simulink model "Microgrid_transition_model_092021"  (R2020a)
settings: Solver=VariableStepAuto  StartTime=0.0  StopTime=10  MaxStep=1e-4  RelTol=1e-3
PreLoadFcn:
  | %run('FC_microgrid_param.m')
  | %load('bat_grid_init.m')
InitFcn:
  | %load myisoModel_init;
  | run('FC_microgrid_param.m')
  | tic
  | run('CARTinitFcn.m')
  | %caseNo = 2;
  | 
  | %if (caseNo == 1)
  | %set_param(['Isolated_grid_paper_model_022521/SignalGen'], 'ActiveScenario', 'PStep222kW');
  | %else
  | %set_param(['Isolated_grid_paper_model_022521/SignalGen'], 'ActiveScenario', 'QStep222kVAr');
  | 
  | %end;
StopFcn:
  | toc
undefined symbols (not defined in the file): breakpoints1, breakpoints2, cp_table_data, ctrl, D1, D11, Delta, DiscIntNeverNeededParam, DT, FC_BESS, find_system, gcbh, libFC_BESS, LowerLimit, magnitude, oversize, pq_ts, sps_rtmsupport, timer, ts, Ts, Ts_APC, Ts_Control, Ts_Power, UpperLimit
libraries: powerlib x128, powerlib_meascontrol x81, simulink x63, powerlib_extras x40, simulink_extras x12, sps_avr x7, pi_ctrl x4, SignalEditorBlockLib x2, libLgBattery x1, libFC_PV x1, eePowerMeasurement x1, spsDieselMotorModel x1
(part 3 of 10)

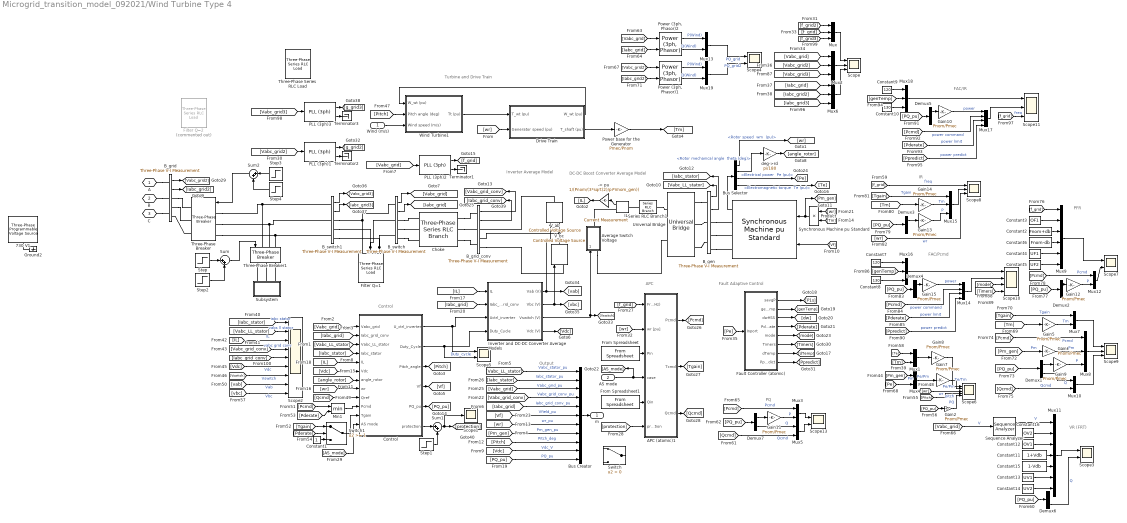
== system Microgrid_transition_model_092021/Wind Turbine Type 4 ==
  note: Control
  note: Turbine and Drive Train
  note: Inverter
      | Average Model
  note: DC-DC Boost Converter
      | Average Model
  note: Fault Adaptive Control
  note: PFR
  note: IR
  note: FAC/Pcmd
  note: PQ
  note: FAC/IR
  note: APC
  note: Output
  note: VR (FRT)
  "Wind (m/s) " : Inport
  AS mode : Inport  Port=2
  -> pu : Gain  Gain=1/(Pnom/(3*sqrt(2)/pi*Vnom_gen))  SaturateOnIntegerOverflow=on  OutDataTypeStr=Inherit: Same as input  ParamDataTypeStr=Inherit: Same as input
  730 V1 : powerlib/Electrical Sources/Three-Phase Programmable Voltage Source  PositiveSequence=[730 0 60]  VariationEntity=None  VariationType=Table of time-amplitude pairs  VariationTypeAlt=Step  VariationStep=-0.2  VariationRate=10  VariationMagnitude=0.3  VariationFrequency=2  VariationTiming=[0.05 0.05+5/60]  VariationPhaseA=off  Amplitudes=[1 1 1.0]  TimeValues=[0 0.03 0.13]  HarmonicGeneration=off  HarmonicA=[1 -0.1 0 2]  HarmonicB=[2 0.15 35 2]*0  Timing="[0.1  2]"  BusType=swing  Pref=0  Qref=0  Qmin=-inf  Qmax=inf
  APC (atomic)1 : Subsystem  TreatAsAtomicUnit=on  SystemSampleTime=0.01
  Average Switch Voltage : Subsystem
  B_gen : powerlib/Measurements/Three-Phase V-I Measurement  VoltageMeasurement=phase-to-phase  SetLabelV=off  LabelV=Vabc  Vpu=on  VpuLL=off  CurrentMeasurement=yes  SetLabelI=off  LabelI=Iabc  Ipu=on  Pbase=Pnom  Vbase=Vnom_gen  OutputType=Complex  PhasorSimulation=off  PSBequivalent=0
      settings: SourceProductBaseCode=MT,PS
  B_grid : powerlib/Measurements/Three-Phase V-I Measurement  VoltageMeasurement=phase-to-ground  SetLabelV=off  LabelV=Vabc  Vpu=on  VpuLL=off  CurrentMeasurement=yes  SetLabelI=off  LabelI=Iabc  Ipu=on  Pbase=Pnom  Vbase=Vnom  OutputType=Complex  PhasorSimulation=off  PSBequivalent=0
      settings: SourceProductBaseCode=MT,PS
  B_grid_conv : powerlib/Measurements/Three-Phase V-I Measurement  VoltageMeasurement=phase-to-ground  SetLabelV=off  LabelV=Vabc  Vpu=on  VpuLL=off  CurrentMeasurement=yes  SetLabelI=off  LabelI=Iabc  Ipu=on  Pbase=Pnom  Vbase=Vnom  OutputType=Complex  PhasorSimulation=off  PSBequivalent=0
      settings: SourceProductBaseCode=MT,PS
  B_switch : powerlib/Measurements/Three-Phase V-I Measurement  VoltageMeasurement=phase-to-ground  SetLabelV=off  LabelV=Vabc  Vpu=on  VpuLL=off  CurrentMeasurement=yes  SetLabelI=off  LabelI=Iabc  Ipu=on  Pbase=Pnom  Vbase=Vnom  OutputType=Complex  PhasorSimulation=off  PSBequivalent=0
      settings: SourceProductBaseCode=MT,PS
  B_switch1 : powerlib/Measurements/Three-Phase V-I Measurement  VoltageMeasurement=phase-to-ground  SetLabelV=off  LabelV=Vabc  Vpu=on  VpuLL=off  CurrentMeasurement=yes  SetLabelI=off  LabelI=Iabc  Ipu=on  Pbase=Pnom  Vbase=Vnom  OutputType=Complex  PhasorSimulation=off  PSBequivalent=0
      settings: SourceProductBaseCode=MT,PS
  Bus Creator : BusCreator  Inputs=11
  Bus Selector : BusSelector  OutputSignals="Mechanical.Rotor speed  wm  (pu),Mechanical.Rotor mechanical angle  theta (deg),Mechanical.Electrical power  Pe (pu),Mechanical.Electromagnetic torque  Te (pu)"
  "Choke " : powerlib/Elements/Three-Phase Series RLC Branch  LConnTagsString=A|B|C  RConnTagsString=A|B|C  BranchType=RL  Resistance=R_RL*Vnom^2/Pnom  Inductance=L_RL*Vnom^2/Pnom/(2*pi*Fnom)  Capacitance=[]  Measurements=None
      settings: SourceProductBaseCode=MT,PS
  Constant1 : Constant
  Constant10 : Constant  Value=130
  Constant11 : Constant  Value=1+Vdb
  Constant12 : Constant  Value=OV1
  Constant13 : Constant  Value=UV1
  Constant14 : Constant  Value=UV2
  Constant15 : Constant  Value=1-Vdb
  Constant16 : Constant  Value=OV2
  Constant2 : Constant  Value=Fnom+db
  Constant3 : Constant  Value=OF1
  Constant4 : Constant  Value=UF1
  Constant5 : Constant  Value=UF2
  Constant6 : Constant  Value=Fnom-db
  Constant7 : Constant  Value=120
  Constant8 : Constant  Value=130
  Constant9 : Constant  Value=120
  Control : Subsystem
  Demux{1..7} (7 alike) : Demux  Outputs=2
  Drive Train : Subsystem  mask(Wind Turbine shaft){H_WT=H_WT/10, Ksh=Ksh, D_mutual=D_mutual, wbase=2*pi*Fnom/p, w_wt0=w_wt0, torque0=torque0, Ts=Ts}
      mask prompts: H_WT "Wind turbine inertia constant H (s):"; Ksh "Shaft spring constant (pu of nominal mechanical torque/rad):"; D_mutual "Shaft mutual damping (pu of nominal mechanical torque/pu dw):"; wbase "Shaft base speed (rad/s):"; w_wt0 "Turbine initial speed (pu of base speed):"; torque0 "Initial output torque (pu of nominal mechanical torque):"; Ts "Sample time (s):"
      mask help:
      | This block implements a wind turbine drive train model. All shaft parameters are referred to high-speed shaft (generator shaft).
      |
      | The first input is the wind turbine torque in per unit (pu) based on the nominal power of the turbine and the base speed of the generator. The second input is the generator speed in pu based on the base speed of the generator.
      |
      | The outputs are:
      | 1- the transmitted torque of the shaft in pu based on the nominal power of the turbine and the base speed of the generator.
      | 2- the wind turbine speed in pu of the base speed of the generator.
  "Fault Controller (atomic) " : Subsystem  TreatAsAtomicUnit=on  SystemSampleTime=Ts_APC
  Filter Q=1 : powerlib/Elements/Three-Phase Series RLC Load  LConnTagsString=A|B|C  Configuration=Y (grounded)  NominalVoltage=Vnom  Vabc=[1e3 1e3 1e3]  Vabcp=[1e3 1e3 1e3]  NominalFrequency=Fnom  UnbalancedPower=off  ActivePower=100  InductivePower=100  CapacitivePower=100  Pabc=[10e3 9e3 11e3]  QLabc=[100 90 110]  QCabc=[100 90 110]  Pabcp=[10e3 9e3 11e3]  QLabcp=[100 90 110]  QCabcp=[100 90 110]  Measurements=None  LoadType=constant Z
      settings: SourceProductBaseCode=MT,PS
  Filter Q=2 : powerlib/Elements/Three-Phase Series RLC Load  Commented=on  LConnTagsString=A|B|C  Configuration=Y (grounded)  NominalVoltage=Vnom  Vabc=[1e3 1e3 1e3]  Vabcp=[1e3 1e3 1e3]  NominalFrequency=Fnom  UnbalancedPower=off  ActivePower=C_var_filter/Q_filter  InductivePower=0  CapacitivePower=C_var_filter  Pabc=[10e3 9e3 11e3]  QLabc=[100 90 110]  QCabc=[100 90 110]  Pabcp=[10e3 9e3 11e3]  QLabcp=[100 90 110]  QCabcp=[100 90 110]  Measurements=None  LoadType=constant Z
      settings: SourceProductBaseCode=MT,PS
  From Spreadsheet : FromSpreadsheet  FileName=Microgrid_cmd.xlsx  SheetName=P  SampleTime=Ts_APC
  From Spreadsheet1 : FromSpreadsheet  FileName=Microgrid_cmd.xlsx  SheetName=Q  SampleTime=Ts_APC
  Gain{2,5..15} (12 alike) : Gain  Gain=Pnom/Pmec
  Ground2 : powerlib/Elements/Ground  LConnTagsString=a
  IL : powerlib/Measurements/Current Measurement  PhasorSimulation=off  OutputType=Complex  PSBequivalent=0
      settings: SourceProductBaseCode=MT,PS
  Inverter and DC-DC Converter Average Models : Subsystem
  Min1 : MinMax  Inputs=2
  Mux{,2,6,8,15..16,18} (7 alike) : Mux  Inputs=3
  Mux{1,3..5,7,10,12..13,19} (9 alike) : Mux  Inputs=2
  Mux11 : Mux  Inputs=7
  Mux14 : Mux
  Mux17 : Mux
  Mux9 : Mux  Inputs=6
  PLL (3ph)1 : powerlib_meascontrol/PLL/PLL (3ph)  Fmin=45  Par_Init=[0, 60]  ParK=[180, 3200, 1]  TcD=1e-4  MaxRateChangeFreq=12  FilterCutOffFreq=25  Ts=Ts  AGC=on
  PLL (3ph)2 : powerlib_meascontrol/PLL/PLL (3ph)  Fmin=45  Par_Init=[0, 60]  ParK=[180, 3200, 1]  TcD=1e-4  MaxRateChangeFreq=12  FilterCutOffFreq=25  Ts=Ts  AGC=on
  PLL (3ph)3 : powerlib_meascontrol/PLL/PLL (3ph)  Fmin=45  Par_Init=[0, 60]  ParK=[180, 3200, 1]  TcD=1e-4  MaxRateChangeFreq=12  FilterCutOffFreq=25  Ts=Ts  AGC=on
  "Power (3ph, Phasor)1" : powerlib_meascontrol/Measurements/Power (3ph, Phasor)
      settings: SourceProductBaseCode=PS
  "Power (3ph, Phasor)2" : powerlib_meascontrol/Measurements/Power (3ph, Phasor)
      settings: SourceProductBaseCode=PS
  Power base for the Generator : Gain  Gain=Pmec/Pnom  SaturateOnIntegerOverflow=on  OutDataTypeStr=Inherit: Same as input  ParamDataTypeStr=Inherit: Same as input
  Product : Product  RndMeth=Zero
  Scope{,8..9,11} (4 alike) : Scope  NumInputPorts=3
  Scope1 : Scope
  Scope10 : Scope  NumInputPorts=4
  Scope{3..5,7,13} (5 alike) : Scope  NumInputPorts=2
  Scope2 : Scope  NumInputPorts=9
  Scope6 : Scope  NumInputPorts=5
  Sequence Analyzer : powerlib_meascontrol/Measurements/Sequence Analyzer  Freq=60  n=1  seq=Positive  InInit=[1, 0]  Ts=Ts
      settings: SourceProductBaseCode=PS
  Series RLC Branch1 : powerlib/Elements/Series RLC Branch  LConnTagsString=__new0  RConnTagsString=__new0  BranchType=RL  Resistance=R_Boost  Inductance=L_Boost  SetiL0=off  InitialCurrent=0  Capacitance=1.0  Setx0=off  InitialVoltage=0  Measurements=Branch current
      settings: SourceProductBaseCode=MT,PS
  Step : Step  Time=4  Before=1  After=0  SampleTime=Ts
  Step1 : Step  Time=99  After=0  SampleTime=Ts
  Step2 : Step  Time=3  SampleTime=Ts
  Step3 : Step  Time=3  Before=1  After=0  SampleTime=Ts
  Step4 : Step  Time=4  SampleTime=Ts
  Subsystem : Subsystem
  Sum : Sum  Inputs=|++
  Sum1 : Sum  Inputs=|++
  Sum2 : Sum  Inputs=|++
  Switch : Switch  Criteria=u2 > Threshold
  Switch1 : Switch  Threshold=1
  Synchronous Machine pu Standard : powerlib/Machines/Synchronous Machine pu Standard  PresetModel=No  MechanicalLoad=Mechanical power Pm  ShowDetailedParameters=on  RotorType=Salient-pole  Units=per unit standard parameters  MeasurementBus=off  NominalParameters="[ Pnom  Vnom_gen Fnom ]"  Reactances1=[ 1.81, 0.3, 0.23, 1.76, 0.65, 0.25, 0.15 ]  Reactances2="[ Xd, Xd1, Xd2, Xq,  Xq2,  Xl ]"  dAxisTimeConstants=Open-circuit  qAxisTimeConstants=Short-circuit  TimeConstants1="[ 4.4849  0.0681  0.1  ]"  TimeConstants2=[ 8.0, 0.03, 1.0, 0.07 ]  TimeConstants3="[  Tdo1  Tdo2  Tq2  ]"  TimeConstants4=[ 8.0, 0.03, 0.3371, 0.0295 ]  TimeConstants5=[ 1.01, 0.053, 0.1 ]  TimeConstants6=[ 1.3201, 0.023, 1.0, 0.07 ]  TimeConstants7="[  1.01  0.053  0.051266  ]"  TimeConstants8=[ 1.3201, 0.0231, 0.3371, 0.0295 ]  StatorResistance=Resistance  Mechanical=[ H F p]  PolePairs=1  InitialConditions=init  SetSaturation=off  Saturation=[0.6404,0.7127,0.8441,0.9214,0.9956,1.082,1.19,1.316,1.457;0.7,0.7698,0.8872,0.9466,0.9969,1.046,1.1,1.151,1.201]  LoadFlowParameters=[1,0,0,0,0]  TsPowergui=0  TsBlock=-1  IterativeModel=Trapezoidal non iterative  IterativeDiscreteModel=Trapezoidal non iterative  BusType=PV  Pref=0  Qref=0  Qmin=-inf  Qmax=inf  PLF=0  QLF=0
      settings: SourceProductBaseCode=MT,PS
  Terminator1 : Terminator
  Terminator2 : Terminator
  Terminator3 : Terminator
  Three-Phase Series RLC Load : powerlib/Elements/Three-Phase Series RLC Load  LConnTagsString=A|B|C  Configuration=Y (grounded)  NominalVoltage=1000  Vabc=[1e3 1e3 1e3]  Vabcp=[1e3 1e3 1e3]  NominalFrequency=60  UnbalancedPower=off  ActivePower=10e3  InductivePower=100  CapacitivePower=100  Pabc=[10e3 9e3 11e3]  QLabc=[100 90 110]  QCabc=[100 90 110]  Pabcp=[10e3 9e3 11e3]  QLabcp=[100 90 110]  QCabcp=[100 90 110]  Measurements=None  LoadType=constant Z
  Three-Phase Breaker : powerlib/Elements/Three-Phase Breaker  InitialState=closed  SwitchA=on  SwitchB=on  SwitchC=on  SwitchTimes=[1000]  External=on  BreakerResistance=Ron_breaker/Nb_WT  SnubberResistance=Rs_breaker/Nb_WT  SnubberCapacitance=Cs_breaker*Nb_WT  Measurements=None
  Three-Phase Breaker1 : powerlib/Elements/Three-Phase Breaker  InitialState=closed  SwitchA=on  SwitchB=on  SwitchC=on  SwitchTimes=[1000]  External=on  BreakerResistance=Ron_breaker/Nb_WT  SnubberResistance=Rs_breaker/Nb_WT  SnubberCapacitance=Cs_breaker*Nb_WT  Measurements=None
  Universal Bridge : powerlib/Power Electronics/Universal Bridge  Arms=3  SnubberResistance=2*Ts_snub/(Pnom/(1000*2*pi*Fnom*Vnom_gen^2))  SnubberCapacitance=Pnom/(1000*2*pi*Fnom*Vnom_gen^2)  Device=Diodes  Ron=1e-6/Nb_wt  Lon=0  ForwardVoltages="[  0  0  ]"  ForwardVoltage=0  GTOparameters=[ 10e-6 , 20e-6 ]  IGBTparameters=[ 1e-6 , 2e-6 ]  Measurements=None  Measurements_2=None  converterType=Rectifier
      settings: SourceProductBaseCode=MT,PS
  V_ab : powerlib/Electrical Sources/Controlled Voltage Source  Initialize=on  Source_Type=AC  Amplitude=0  Phase=0  Frequency=0  Measurements=None
      settings: SourceProductBaseCode=MT,PS
  V_bc : powerlib/Electrical Sources/Controlled Voltage Source  Initialize=on  Source_Type=AC  Amplitude=0  Phase=0  Frequency=0  Measurements=None
      settings: SourceProductBaseCode=MT,PS
  Wind Turbine1 : Subsystem  mask(Wind Turbine){Prated=Pmec, c1_c8=c1_c8, K1_K2=K1_K2, wind0=wind0, Ts=Ts}
      mask prompts: Prated "Nominal mechanical output power (W):"; c1_c8 "Coefficients [c1 ... c8]"; K1_K2 "Parameters [K1 K2]"; wind0 "Initial wind speed (m/s):"; Ts "Sample time (s):"
      mask help:
      | This block implements a generic wind turbine models.
      |
      | The first input is the turbine speed in per unit of the generator base speed. For a synchronous or asynchronous generator, the base speed is the synchronous speed. For a permanent-magnet generator, the base speed is defined as the speed producing nominal voltage at  no load. The second input is the blade pitch angle in degrees. The third input is the wind speed in m/s.
      |
      | The output is the torque applied to the drive train in per unit based on the nominal power of the turbine and the base speed of the generator.
      mask init:
      | c1 = c1_c8(1);
      | c2 = c1_c8(2);
      | c3 = c1_c8(3);
      | c4 = c1_c8(4);
      | c5 = c1_c8(5);
      | c6 = c1_c8(6);
      | c7 = c1_c8(7);;
      | c8 = c1_c8(8);
      | 
      | K1=K1_K2(1);
      | K2=K1_K2(2);
      settings: OpenFcn=power_openblockproxy();
      mask Display: disp('');
  deg->rd : Gain  Gain=pi/180  SaturateOnIntegerOverflow=on  OutDataTypeStr=Inherit: Same as input  ParamDataTypeStr=Inherit: Same as input
  A : PMIOPort  Tag=PMCPort  Side=Left
  B : PMIOPort  Tag=PMCPort  Port=2  Side=Left
  C : PMIOPort  Tag=PMCPort  Port=3  Side=Left
  m : Outport  VectorParamsAs1DForOutWhenUnconnected=off
  wires:
  Bus Selector/2 -> deg->rd/1  "<Rotor mechanical angle  theta (deg)>"
  deg->rd/1 -> [angle_rotor]
  Bus Selector/1 -> [wr]  "<Rotor speed  wm  (pu)>"
  [Iabc_grid] -> Inverter and DC-DC Converter Average Models/2(Iabc_grid_conv)
  [IL] -> Inverter and DC-DC Converter Average Models/1(IL)
  [Vabc_grid] -> Control/1(Vabc_grid)
  [Iabc_grid] -> Control/2(Iabc_grid_conv)
  [Vabc_LL_stator] -> Control/3(Vabc_LL_stator)
  [Iabc_stator] -> Control/4(Iabc_stator)
  [Vdc] -> Control/6(Vdc)
  [angle_rotor] -> Control/7(angle_rotor)
  [wr] -> Control/8(wr)
  Control/2(Duty_Cycle) -> Scope5/2, Inverter and DC-DC Converter Average Models/4(Duty_Cycle)  "Duty_cycle"
  Control/3(Pitch_angle) -> [Pitch]
  Control/4(Vf) -> [Vf]
  Control/5(PQ_pu) -> [PQ_pu]
  [IL] -> Control/5(IL)
  Control/1(U_ctrl_inverter) -> Scope5/1, Inverter and DC-DC Converter Average Models/3(Uctrl_inverter)
  Inverter and DC-DC Converter Average Models/4(Vdc (V)) -> [Vdc]
  [Qcmd] -> Control/9(Qref)
  [Pitch] -> Wind Turbine1/2(Pitch angle (deg))
  Drive Train/2(T_shaft (pu)) -> Power base for the Generator/1
  Drive Train/1(W_wt (pu)) -> Wind Turbine1/1(W_wt (pu))
  "Wind (m/s) "/1 -> Wind Turbine1/3(Wind speed (m/s))
  Power base for the Generator/1 -> [Tm]
  [wr] -> Drive Train/2(Generator speed (pu))
  Wind Turbine1/1(Tt (pu)) -> Drive Train/1(T_wt (pu))
  Bus Selector/4 -> [Te]  "<Electromagnetic torque  Te (pu)>"
  Bus Selector/3 -> [Pe]  "<Electrical power  Pe (pu)>"
  Inverter and DC-DC Converter Average Models/1(Vab (V)) -> V_ab/1, [vab]
  [wr] -> Product/1
  B_gen/2 -> [Iabc_stator]
  Inverter and DC-DC Converter Average Models/2(Vbc (V)) -> V_bc/1, [vbc]
  B_switch/2 -> [Iabc_grid]
  Synchronous Machine pu Standard/1 -> Bus Selector/1
  B_switch/1 -> [Vabc_grid]
  [Tm] -> Product/2
  IL/1 -> -> pu/1
  B_gen/1 -> [Vabc_LL_stator]
  [Vf] -> Synchronous Machine pu Standard/2
  Inverter and DC-DC Converter Average Models/3(Vswitch (V)) -> Average Switch Voltage/1(Vswitch), [Vswitch]
  B_grid_conv/1 -> [Vabc_grid_conv]
  Product/1 -> Synchronous Machine pu Standard/1, [Pm_gen]
  -> pu/1 -> [IL]
  Control/6(protection) -> Sum1/1
  "Fault Controller (atomic) "/1(savgP) -> [P1s]
  [Pe] -> "Fault Controller (atomic) "/1(Inport)
  "Fault Controller (atomic) "/8(Ppredict) -> [Ppredict]
  "Fault Controller (atomic) "/2(genTemp) -> [genTemp]
  "Fault Controller (atomic) "/7(dTemp) -> [dTemp]
  "Fault Controller (atomic) "/6(Timers) -> [Timers]
  "Fault Controller (atomic) "/4(Pderate) -> [Pderate]
  "Fault Controller (atomic) "/3(dwHSS) -> [dw]
  "Fault Controller (atomic) "/5(mode) -> [mode]
  Gain8/1 -> Scope6/1  "Te/Tm"
  [Tm] -> Gain14/1
  [PQ_pu] -> Demux2/1
  [Tm] -> Mux1/2
  Constant10/1 -> Mux18/3
  [Qcmd] -> Mux10/2  "Qcmd"
  Mux12/1 -> Scope7/2
  [Pcmd] -> Mux8/1  "Pcmd"
  [Te] -> Mux1/1
  Mux9/1 -> Scope7/1
  [PQ_pu] -> Demux4/1
  Gain13/1 -> Mux15/3  "P"
  Gain14/1 -> Mux15/2  "Tm"
  Gain12/1 -> Mux12/2  "P"
  [Tgain] -> Mux7/1  "Tgain"
  Demux5/1 -> Gain10/1
  Gain9/1 -> Mux8/3  "P"
  [Pderate] -> Mux14/3  "power limit"
  [Pe] -> Mux4/2
  [wr] -> Scope8/3  "wr"
  Mux17/1 -> Scope11/2
  Demux1/1 -> Gain9/1
  [Timers] -> Scope10/4
  Mux5/1 -> Scope13/2
  Mux4/1 -> Gain7/1  "Pe/Pm"
  [f_grid] -> Scope8/1  "freq"
  [Ppredict] -> Mux14/4  "power predict"
  Mux10/1 -> Scope9/3
  Demux1/2 -> Mux10/1  "Q"
  [Pm_gen] -> Mux4/1  "Pm"
  [genTemp] -> Mux18/2
  [Pitch] -> Scope6/4  "pitch"
  Mux14/1 -> Scope10/2
  [PQ_pu] -> Gain2/1
  Constant9/1 -> Mux18/1
  Constant8/1 -> Mux16/3
  [PQ_pu] -> Demux1/1
  [Pderate] -> Mux17/3  "power limit"
  [Pcmd] -> Mux17/2  "power command"
  Mux1/1 -> Gain8/1
  Mux8/1 -> Scope9/2
  Gain15/1 -> Mux14/1  "power"
  Constant2/1 -> Mux9/3
  Mux16/1 -> Scope10/1
  [Pcmd] -> Mux14/2  "power command"
  [Pcmd] -> Mux12/1  "Pcmd"
  Constant7/1 -> Mux16/1
  Mux15/1 -> Scope8/2
  [PQ_pu] -> Demux5/1
  Gain11/1 -> Mux3/2  "P"
  Gain5/1 -> Mux7/2  "Tm"
  [Pm_gen] -> Gain6/1  "Pm"
  [PQ_pu] -> Demux7/1
  [f_grid] -> Scope11/3  "freq"
  Gain10/1 -> Mux17/1  "power"
  [Tgain] -> Mux15/1  "Tgain"
  Gain6/1 -> Mux8/2  "Pm"
  [Qcmd] -> Mux5/2  "Qcmd"
  [Tm] -> Gain5/1
  [wr] -> Scope6/3  "wr"
  Mux3/1 -> Scope13/1
  Demux2/1 -> Gain12/1
  Demux4/1 -> Gain15/1
  Constant3/1 -> Mux9/2
  Constant5/1 -> Mux9/6
  Demux7/2 -> Mux5/1  "Q"
  [PQ_pu] -> Demux3/1
  [Pcmd] -> Mux3/1  "Pcmd"
  [Ppredict] -> Mux17/4  "power predict"
  Constant6/1 -> Mux9/4
  Demux3/1 -> Gain13/1
  Constant4/1 -> Mux9/5
  Gain2/1 -> Scope6/5  "PQ"
  Demux7/1 -> Gain11/1
  Mux18/1 -> Scope11/1
  Mux7/1 -> Scope9/1
  [f_grid] -> Mux9/1
  Gain7/1 -> Scope6/2  "Pe/Pm"
  [mode] -> Scope10/3
  [genTemp] -> Mux16/2
  [Pderate] -> Min1/2
  [Pcmd] -> Min1/1
  Min1/1 -> Control/10(Pcmd)
  [Pderate] -> Switch1/2
  Switch1/1 -> Control/11(Tgain)
  Constant1/1 -> Switch1/3
  [Tgain] -> Switch1/1
  PLL (3ph)2/2 -> Terminator1/1
  [Vabc_grid] -> PLL (3ph)2/1
  PLL (3ph)2/1 -> [f_grid]
  From Spreadsheet1/1 -> APC (atomic)1/5(Qin)
  [f_grid] -> APC (atomic)1/1(Freq (Hz))
  APC (atomic)1/3(Qcmd) -> [Qcmd]
  APC (atomic)1/2(Tcmd) -> [Tgain]
  [protection] -> APC (atomic)1/6(protection)
  [wr] -> APC (atomic)1/2(wr [pu])
  AS mode/1 -> APC (atomic)1/4(case), [AS_mode]
  APC (atomic)1/1(Pcmd) -> [Pcmd]
  From Spreadsheet/1 -> APC (atomic)1/3(Pin)
  [AS_mode] -> Control/12(AS mode)
  [Pm_gen] -> Bus Creator/8  "Pm_gen_pu"
  Bus Creator/1 -> m/1
  [Iabc_grid] -> Bus Creator/5  "Iabc_grid_conv_pu"
  [Pitch] -> Bus Creator/9  "Pitch_deg"
  [PQ_pu] -> Bus Creator/11  "PQ_pu"
  [Vf] -> Bus Creator/6  "Vfield_pu"
  [Vdc] -> Bus Creator/10  "Vdc_V"
  [Vabc_LL_stator] -> Bus Creator/1  "Vabc_stator_pu"
  [Vabc_grid] -> Bus Creator/3  "Vabc_grid_pu"
  [Iabc_stator] -> Bus Creator/2  "Iabc_stator_pu"
  [wr] -> Bus Creator/7  "wr_pu"
  [Vabc_grid_conv] -> Bus Creator/4  "Vabc_grid_conv_pu"
  B_grid/2 -> [Iabc_grid2]
  B_grid/1 -> [Vabc_grid2]
  PLL (3ph)1/1 -> [g_grid2]
  PLL (3ph)1/2 -> Terminator2/1
  [Vabc_grid2] -> PLL (3ph)1/1
  [f_grid2] -> Mux/1
  [f_grid] -> Mux/2
  [Vabc_grid] -> Mux2/1
  [Vabc_grid2] -> Mux2/2
  Mux2/1 -> Scope/2
  Mux/1 -> Scope/1
  Sum2/1 -> Three-Phase Breaker/1
  Step1/1 -> Sum1/2
  Sum1/1 -> [protection], Scope1/1
  [Iabc_stator] -> Scope2/1  "iabc stator"
  [Vabc_LL_stator] -> Scope2/2  "vabs ll stator"
  [IL] -> Scope2/3  "IL"
  [Vabc_grid_conv] -> Scope2/4  "vabc grid conv"
  [Vdc] -> Scope2/6  "Vdc"
  [Vswitch] -> Scope2/7  "Vswitch"
  [vab] -> Scope2/8  "Vab"
  [vbc] -> Scope2/9  "Vbc"
  Sequence Analyzer/1 -> Mux11/1  "V"
  Constant13/1 -> Mux11/6
  Constant15/1 -> Mux11/5
  Constant14/1 -> Mux11/7
  Constant12/1 -> Mux11/3
  Constant11/1 -> Mux11/4
  Mux11/1 -> Scope3/1
  [Vabc_grid] -> Sequence Analyzer/1  "V"
  Constant16/1 -> Mux11/2
  Demux6/2 -> Scope3/2  "Q"
  [PQ_pu] -> Demux6/1
  "Power (3ph, Phasor)2"/2 -> Mux13/2  "Q(Wind)"
  [Vabc_grid] -> "Power (3ph, Phasor)2"/1
  "Power (3ph, Phasor)2"/1 -> Mux13/1  "P(Wind)"
  [Iabc_grid] -> "Power (3ph, Phasor)2"/2
  Mux13/1 -> Scope4/1  "PQ_grid"
  Mux19/1 -> Scope4/2  "PQ_grid2"
  [Iabc_grid2] -> "Power (3ph, Phasor)1"/2
  [Vabc_grid2] -> "Power (3ph, Phasor)1"/1
  "Power (3ph, Phasor)1"/1 -> Mux19/1  "P(Wind)"
  "Power (3ph, Phasor)1"/2 -> Mux19/2  "Q(Wind)"
  B_switch1/1 -> [Vabc_grid3]
  B_switch1/2 -> [Iabc_grid3]
  PLL (3ph)3/1 -> [g_grid3]
  PLL (3ph)3/2 -> Terminator3/1
  [Vabc_grid3] -> PLL (3ph)3/1
  [f_grid3] -> Mux/3
  [Vabc_grid3] -> Mux2/3
  [Iabc_grid] -> Mux6/1
  [Iabc_grid2] -> Mux6/2
  [Iabc_grid3] -> Mux6/3
  Mux6/1 -> Scope/3
  B_grid_conv/2 -> [Iabc_grid_conv]
  [Iabc_grid_conv] -> Scope2/5
  Step2/1 -> Sum/2
  Step/1 -> Sum/1
  Sum/1 -> Three-Phase Breaker1/1
  Step4/1 -> Sum2/2
  Step3/1 -> Sum2/1
  connections:
  B_grid/RConn1 -- Three-Phase Breaker/RConn1
  B_grid/RConn2 -- Three-Phase Breaker/RConn2
  Three-Phase Breaker/RConn3 -- B_grid/RConn3
  B_grid_conv/RConn2 -- V_bc/RConn1 -- V_ab/LConn1
  Filter Q=1/LConn3 -- B_switch/LConn3 -- B_switch1/RConn3
  Filter Q=1/LConn2 -- B_switch/LConn2 -- B_switch1/RConn2
  B_switch/LConn1 -- B_switch1/RConn1 -- Filter Q=1/LConn1
  B_switch/RConn3 -- "Choke "/LConn3
  "Choke "/RConn3 -- B_grid_conv/LConn3
  B_switch/RConn2 -- "Choke "/LConn2
  Universal Bridge/LConn1 -- B_gen/LConn1
  B_gen/RConn2 -- Synchronous Machine pu Standard/RConn2
  Average Switch Voltage/RConn1 -- IL/RConn1
  Universal Bridge/LConn2 -- B_gen/LConn2
  Universal Bridge/LConn3 -- B_gen/LConn3
  V_ab/RConn1 -- B_grid_conv/RConn1
  B_switch/RConn1 -- "Choke "/LConn1
  B_gen/RConn1 -- Synchronous Machine pu Standard/RConn1
  "Choke "/RConn1 -- B_grid_conv/LConn1
  "Choke "/RConn2 -- B_grid_conv/LConn2
  B_grid_conv/RConn3 -- V_bc/LConn1
  Series RLC Branch1/LConn1 -- Universal Bridge/RConn1
  B_gen/RConn3 -- Synchronous Machine pu Standard/RConn3
  Series RLC Branch1/RConn1 -- IL/LConn1
  Average Switch Voltage/LConn1 -- Universal Bridge/RConn2
  A/RConn1 -- B_grid/LConn1
  B/RConn1 -- B_grid/LConn2
  C/RConn1 -- B_grid/LConn3
  Three-Phase Breaker/LConn1 -- Three-Phase Breaker1/LConn1 -- B_switch1/LConn1
  Three-Phase Breaker/LConn2 -- Three-Phase Breaker1/LConn2 -- B_switch1/LConn2
  Three-Phase Breaker/LConn3 -- Three-Phase Breaker1/LConn3 -- B_switch1/LConn3
  Subsystem/RConn3 -- Three-Phase Breaker1/RConn3
  Subsystem/RConn2 -- Three-Phase Breaker1/RConn2
  Subsystem/RConn1 -- Three-Phase Breaker1/RConn1
  Ground2/LConn1 -- 730 V1/LConn1

== system Microgrid_transition_model_092021/../Average Switch Voltage ==
  Vswitch : Inport
  Diode : powerlib/Power Electronics/Diode  Ron=1e-6/Nb_wt  Lon=0  Vf=0  IC=0  UseSnubber=off  Rs=1e5  Cs=inf  Measurements=off
      settings: SourceProductBaseCode=MT,PS
  V : powerlib/Electrical Sources/Controlled Voltage Source  Initialize=on  Source_Type=AC  Amplitude=0  Phase=0  Frequency=0  Measurements=None
      settings: SourceProductBaseCode=MT,PS
  + : PMIOPort  Side=Right
  - : PMIOPort  Port=2  Side=Left
  wires:
  Vswitch/1 -> V/1
  connections:
  -/RConn1 -- V/LConn1
  +/RConn1 -- Diode/LConn1
  Diode/RConn1 -- V/RConn1

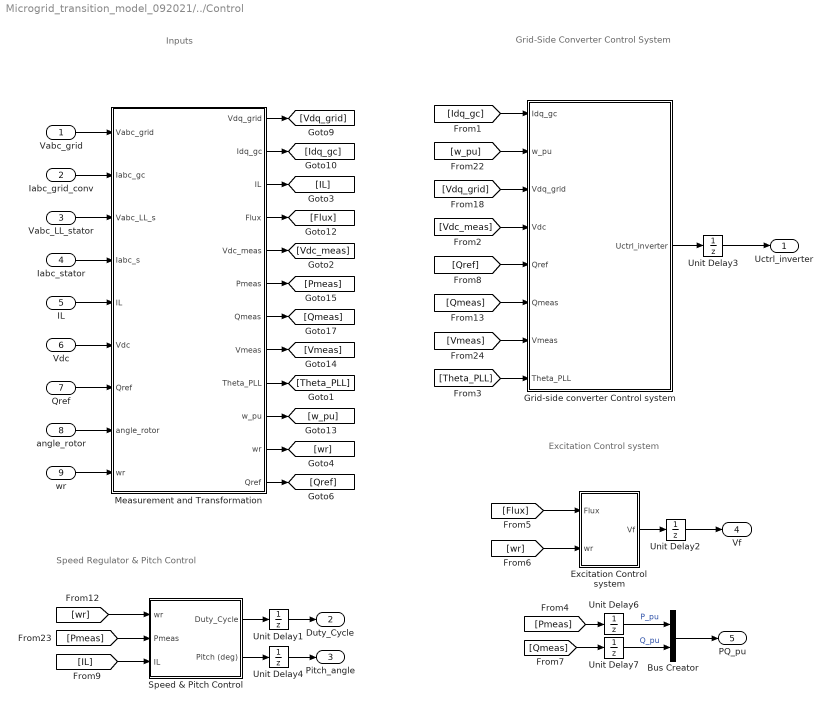
== system Microgrid_transition_model_092021/../Control ==
  note: Excitation
      | Control system
  note: Speed Regulator & Pitch Control
  note: Grid-Side Converter
      | Control System
  note: Inputs
  Vabc_grid : Inport
  Iabc_grid_conv : Inport  Port=2
  Vabc_LL_stator : Inport  Port=3
  Iabc_stator : Inport  Port=4
  IL : Inport  Port=5
  Vdc : Inport  Port=6
  Qref : Inport  Port=7
  angle_rotor : Inport  Port=8
  wr : Inport  Port=9
  Bus Creator : BusCreator  Inputs=2
  Excitation Control system : Subsystem
  Grid-side converter Control system : Subsystem
  Measurement and Transformation : Subsystem
  Speed & Pitch Control : Subsystem
  Unit Delay{1..4,6..7} (6 alike) : UnitDelay  SampleTime=Ts  HasFrameUpgradeWarning=on
  Uctrl_inverter : Outport  VectorParamsAs1DForOutWhenUnconnected=off
  Duty_Cycle : Outport  Port=2  VectorParamsAs1DForOutWhenUnconnected=off
  Pitch_angle : Outport  Port=3  VectorParamsAs1DForOutWhenUnconnected=off
  Vf : Outport  Port=4  VectorParamsAs1DForOutWhenUnconnected=off
  PQ_pu : Outport  Port=5  VectorParamsAs1DForOutWhenUnconnected=off
  wires:
  [IL] -> Speed & Pitch Control/3(IL)
  IL/1 -> Measurement and Transformation/5(IL)
  Measurement and Transformation/3("IL ") -> [IL]
  Unit Delay7/1 -> Bus Creator/2  "Q_pu"
  Unit Delay6/1 -> Bus Creator/1  "P_pu"
  [Qmeas] -> Unit Delay7/1
  [Pmeas] -> Unit Delay6/1
  Unit Delay4/1 -> Pitch_angle/1
  Unit Delay1/1 -> Duty_Cycle/1
  Unit Delay2/1 -> Vf/1
  Unit Delay3/1 -> Uctrl_inverter/1
  Bus Creator/1 -> PQ_pu/1
  Measurement and Transformation/9(Theta_PLL) -> [Theta_PLL]
  [Theta_PLL] -> Grid-side converter Control system/8(Theta_PLL)
  Grid-side converter Control system/1(Uctrl_inverter) -> Unit Delay3/1
  wr/1 -> Measurement and Transformation/9(wr)
  angle_rotor/1 -> Measurement and Transformation/8(angle_rotor)
  Qref/1 -> Measurement and Transformation/7(Qref)
  Vdc/1 -> Measurement and Transformation/6(Vdc)
  Iabc_stator/1 -> Measurement and Transformation/4(Iabc_s)
  Vabc_LL_stator/1 -> Measurement and Transformation/3(Vabc_LL_s)
  Iabc_grid_conv/1 -> Measurement and Transformation/2(Iabc_gc)
  Vabc_grid/1 -> Measurement and Transformation/1(Vabc_grid)
  [wr] -> Excitation Control system/2(wr)
  [Flux] -> Excitation Control system/1(Flux)
  Measurement and Transformation/4(Flux) -> [Flux]
  Speed & Pitch Control/1(Duty_Cycle) -> Unit Delay1/1
  [Pmeas] -> Speed & Pitch Control/2(Pmeas)
  [wr] -> Speed & Pitch Control/1(wr)
  [Vmeas] -> Grid-side converter Control system/7(Vmeas)
  [Qmeas] -> Grid-side converter Control system/6(Qmeas)
  [Qref] -> Grid-side converter Control system/5(Qref)
  Measurement and Transformation/12("Qref ") -> [Qref]
  Measurement and Transformation/11("wr ") -> [wr]
  Measurement and Transformation/5(Vdc_meas) -> [Vdc_meas]
  [Vdc_meas] -> Grid-side converter Control system/4(Vdc)
  [Vdq_grid] -> Grid-side converter Control system/3(Vdq_grid)
  [w_pu] -> Grid-side converter Control system/2(w_pu)
  [Idq_gc] -> Grid-side converter Control system/1(Idq_gc)
  Measurement and Transformation/10(w_pu) -> [w_pu]
  Measurement and Transformation/8(Vmeas) -> [Vmeas]
  Measurement and Transformation/6(Pmeas) -> [Pmeas]
  Measurement and Transformation/2(Idq_gc) -> [Idq_gc]
  Measurement and Transformation/1(Vdq_grid) -> [Vdq_grid]
  Measurement and Transformation/7(Qmeas) -> [Qmeas]
  Speed & Pitch Control/2(Pitch (deg)) -> Unit Delay4/1
  Excitation Control system/1(Vf) -> Unit Delay2/1

== system Microgrid_transition_model_092021/../Drive Train ==
  note: Shaft
  note: Turbine
  note: Wind turbine drive train based on a 2-masse model
  T_wt (pu) : Inport
  Generator speed (pu) : Inport  Port=2
  1_2H_WT : Gain  Gain=1/(2*H_WT)  SaturateOnIntegerOverflow=on  OutDataTypeStr=Inherit: Same as input  ParamDataTypeStr=Inherit: Same as input
  Discrete-Time Integrator : DiscreteIntegrator  InitialCondition=w_wt0  SampleTime=Ts  ICPrevOutput=DiscIntNeverNeededParam  ICPrevScaledInput=DiscIntNeverNeededParam
  Discrete-Time Integrator1 : DiscreteIntegrator  InitialCondition=torque0/Ksh  SampleTime=Ts  ICPrevOutput=DiscIntNeverNeededParam  ICPrevScaledInput=DiscIntNeverNeededParam
  Mutual damping : Gain  Gain=D_mutual  SaturateOnIntegerOverflow=on  OutDataTypeStr=Inherit: Same as input  ParamDataTypeStr=Inherit: Same as input
  Stiffness : Gain  Gain=Ksh  SaturateOnIntegerOverflow=on  OutDataTypeStr=Inherit: Same as input  ParamDataTypeStr=Inherit: Same as input
  Sum : Sum  Inputs=+-  InputSameDT=on  SaturateOnIntegerOverflow=on  OutDataTypeStr=Inherit: Same as first input
  Sum1 : Sum  Inputs=+-  InputSameDT=on  SaturateOnIntegerOverflow=on  OutDataTypeStr=Inherit: Same as first input
  Sum2 : Sum  InputSameDT=on  SaturateOnIntegerOverflow=on  OutDataTypeStr=Inherit: Same as first input
  wbase : Gain  Gain=wbase  SaturateOnIntegerOverflow=on  OutDataTypeStr=Inherit: Same as input  ParamDataTypeStr=Inherit: Same as input
  W_wt (pu) : Outport  VectorParamsAs1DForOutWhenUnconnected=off
  T_shaft (pu) : Outport  Port=2  VectorParamsAs1DForOutWhenUnconnected=off
  wires:
  wbase/1 -> Discrete-Time Integrator1/1
  Discrete-Time Integrator1/1 -> Stiffness/1
  Stiffness/1 -> Sum2/1
  Sum/1 -> 1_2H_WT/1
  1_2H_WT/1 -> Discrete-Time Integrator/1
  Discrete-Time Integrator/1 -> Sum1/1, W_wt (pu)/1
  Generator speed (pu)/1 -> Sum1/2
  Sum1/1 -> wbase/1, Mutual damping/1
  Mutual damping/1 -> Sum2/2
  Sum2/1 -> Sum/2, T_shaft (pu)/1
  T_wt (pu)/1 -> Sum/1

== system Microgrid_transition_model_092021/../Inverter and DC-DC Converter Average Models ==
  note: Current of the boost converter diode
      | This diode is not illustrated in the average model
  note: Inverter and DC-DC Boost Converter
      | Average Models
  note: DC-DC Converter
      | Average Model
  note: Vab Vbc Inverter
      | Average Model
  note: Pac=Vab*Ia -Vbc*Ic
      | Pdc=Vdc*Idc
  IL : Inport
  Iabc_grid_conv : Inport  Port=2
  Uctrl_inverter : Inport  Port=3
  Duty_Cycle : Inport  Port=4
  0.1 : Gain  Gain=0.5
  0.2 : Gain  Gain=-1
  0.5 : Gain  Gain=0.5
  1/C : Gain  Gain=1/C_DClink
  Constant2 : Constant
  Demux : Demux  Outputs=3
  Demux2 : Demux  Outputs=3
  Discrete-Time Integrator : DiscreteIntegrator  InitialCondition=Vdc_nom  SampleTime=Ts  LimitOutput=on  LowerSaturationLimit=eps  ICPrevOutput=DiscIntNeverNeededParam  ICPrevScaledInput=DiscIntNeverNeededParam
  Product{1..4,6..7} (6 alike) : Product  RndMeth=Zero
  Product5 : Product  Inputs=*/  RndMeth=Zero
  Saturation Dynamic : simulink/Discontinuities/Saturation Dynamic  OutMin=[]  OutMax=[]  OutDataTypeStr=Inherit: Same as second input  OutDataType=sfix(16)  OutScaling=2^-10  DoSatur=off
  Saturation Dynamic1 : simulink/Discontinuities/Saturation Dynamic  OutMin=[]  OutMax=[]  OutDataTypeStr=Inherit: Same as second input  OutDataType=sfix(16)  OutScaling=2^-10  DoSatur=off
  Subtract1 : Sum  Inputs=+-
  Subtract2 : Sum  Inputs=+-
  Subtract3 : Sum  Inputs=+-
  Subtract4 : Sum
  Sum : Sum  Inputs=|+-
  Terminator : Terminator
  pu->A : Gain  Gain=Pnom/(3*sqrt(2)/pi*Vnom_gen)  SaturateOnIntegerOverflow=on  OutDataTypeStr=Inherit: Same as input  ParamDataTypeStr=Inherit: Same as input
  "pu->A " : Gain  Gain=Pnom/sqrt(3)/Vnom*sqrt(2)  SaturateOnIntegerOverflow=on  OutDataTypeStr=Inherit: Same as input  ParamDataTypeStr=Inherit: Same as input
  Vab (V) : Outport  VectorParamsAs1DForOutWhenUnconnected=off
  Vbc (V) : Outport  Port=2  VectorParamsAs1DForOutWhenUnconnected=off
  Vswitch (V) : Outport  Port=3  VectorParamsAs1DForOutWhenUnconnected=off
  Vdc (V) : Outport  Port=4  VectorParamsAs1DForOutWhenUnconnected=off
  wires:
  pu->A/1 -> Product2/2
  [Idiode] -> Subtract4/1  "Idiode"
  Saturation Dynamic1/1 -> [Vbc], Vbc (V)/1
  Saturation Dynamic/1 -> [Vab], Vab (V)/1
  Uctrl_inverter/1 -> Demux2/1
  0.2/1 -> Saturation Dynamic1/3, Saturation Dynamic/3
  0.1/1 -> Saturation Dynamic1/2  "Vbc_avg"
  0.5/1 -> Saturation Dynamic/2  "Vab_avg"
  Demux2/1 -> Subtract3/1
  Demux2/2 -> Subtract1/1, Subtract3/2
  Demux2/3 -> Subtract1/2
  Product6/1 -> 0.5/1
  Product7/1 -> 0.1/1
  Subtract3/1 -> Product6/1
  Subtract1/1 -> Product7/1
  [Vdc] -> Product7/2, Product6/2, Saturation Dynamic/1, Saturation Dynamic1/1, 0.2/1
  Product5/1 -> Subtract4/2  "Idc grid converter"
  [Vbc] -> Product4/1
  [Vab] -> Product3/1
  Demux/3 -> Product4/2  "Ic"
  Subtract2/1 -> Product5/1  "Pac"
  Product3/1 -> Subtract2/1
  Product4/1 -> Subtract2/2
  Duty_Cycle/1 -> Sum/2
  Iabc_grid_conv/1 -> "pu->A "/1
  Demux/2 -> Terminator/1
  "pu->A "/1 -> Demux/1
  Demux/1 -> Product3/2  "Ia"
  Subtract4/1 -> 1/C/1
  Discrete-Time Integrator/1 -> [Vdc], Product5/2, Vdc (V)/1
  1/C/1 -> Discrete-Time Integrator/1
  Constant2/1 -> Sum/1
  Sum/1 -> Product1/2, Product2/1
  IL/1 -> pu->A/1
  [Vdc] -> Product1/1
  Product2/1 -> [Idiode]
  Product1/1 -> Vswitch (V)/1

== system Microgrid_transition_model_092021/../Wind Turbine1 ==
  W_wt (pu) : Inport
  Pitch angle (deg) : Inport  Port=2
  Wind speed (m/s) : Inport  Port=3
  ->pu : Gain  Gain=1/Prated
  2-D Lookup Table1 : Lookup_n-D  BreakpointsForDimension1=breakpoints1  BreakpointsForDimension2=breakpoints2  Table=cp_table_data  InternalRulePriority=Speed  RndMeth=Simplest  InputSameDT=on
  Avoid div. by zero : Saturate  UpperLimit=inf  LowerLimit=eps
  "Avoid div. by zero " : Saturate  UpperLimit=inf  LowerLimit=eps
  Fcn1 : Fcn  Expr=K1*u[2]/u[1]
  Fcn2 : Fcn  Commented=on  Expr=c1*(c6*u[1] + (-c4 - c3*(2.5 + u[2]) + c2*(1/(u[1] + c7*(2.5 + u[2])) -c8/(1 + (2.5 + u[2])^3)))/exp(c5*(1/(u[1] + c7*(2.5 + u[2])) - c8/(1 + (2.5 + u[2])^3))))
  "K2*Cp*wind^3 " : Fcn  Expr=K2*u[1]^3*u[2]
  Mux : Mux  Inputs=2
  Mux2 : Mux  Inputs=2
  Product2 : Product  Inputs=*/  InputSameDT=on  SaturateOnIntegerOverflow=on  OutDataTypeStr=Inherit: Same as first input
  Tt (pu) : Outport  VectorParamsAs1DForOutWhenUnconnected=off
  wires:
  "K2*Cp*wind^3 "/1 -> ->pu/1
  "Avoid div. by zero "/1 -> Product2/2, Mux/2
  Avoid div. by zero/1 -> Mux/1, Mux2/1
  W_wt (pu)/1 -> "Avoid div. by zero "/1
  Pitch angle (deg)/1 -> 2-D Lookup Table1/2
  Mux2/1 -> "K2*Cp*wind^3 "/1
  2-D Lookup Table1/1 -> Mux2/2  "Cp"
  Mux/1 -> Fcn1/1
  Fcn1/1 -> 2-D Lookup Table1/1  "lambda"
  Wind speed (m/s)/1 -> Avoid div. by zero/1
  Product2/1 -> Tt (pu)/1
  ->pu/1 -> Product2/1  "power_pu"

== system Microgrid_transition_model_092021/../Wind Turbine2 ==
  W_wt (pu) : Inport
  Pitch angle (deg) : Inport  Port=2
  Wind speed (m/s) : Inport  Port=3
  ->pu : Gain  Gain=1/Prated
  Avoid div. by zero : Saturate  UpperLimit=inf  LowerLimit=eps
  "Avoid div. by zero " : Saturate  UpperLimit=inf  LowerLimit=eps
  Fcn1 : Fcn  Expr=K1*u[2]/u[1]
  Fcn2 : Fcn  Expr=c1*(c6*u[1] + (-c4 - c3*(2.5 + u[2]) + c2*(1/(u[1] + c7*(2.5 + u[2])) -c8/(1 + (2.5 + u[2])^3)))/exp(c5*(1/(u[1] + c7*(2.5 + u[2])) - c8/(1 + (2.5 + u[2])^3))))
  "K2*Cp*wind^3 " : Fcn  Expr=K2*u[1]^3*u[2]
  Mux : Mux  Inputs=2
  Mux1 : Mux  Inputs=2
  Mux2 : Mux  Inputs=2
  Product2 : Product  Inputs=*/  InputSameDT=on  SaturateOnIntegerOverflow=on  OutDataTypeStr=Inherit: Same as first input
  Tt (pu) : Outport  VectorParamsAs1DForOutWhenUnconnected=off
  wires:
  ->pu/1 -> Product2/1  "power_pu"
  Product2/1 -> Tt (pu)/1
  Wind speed (m/s)/1 -> Avoid div. by zero/1
  Fcn1/1 -> Mux1/1  "lambda"
  Mux1/1 -> Fcn2/1
  Mux/1 -> Fcn1/1
  Fcn2/1 -> Mux2/2  "Cp"
  Mux2/1 -> "K2*Cp*wind^3 "/1
  Pitch angle (deg)/1 -> Mux1/2
  W_wt (pu)/1 -> "Avoid div. by zero "/1
  Avoid div. by zero/1 -> Mux2/1, Mux/1
  "Avoid div. by zero "/1 -> Mux/2, Product2/2
  "K2*Cp*wind^3 "/1 -> ->pu/1

== system Microgrid_transition_model_092021/Defferable Load (0-446.25 kW)/Resistive Loads ==
  Bit 0 : powerlib/Elements/Three-Phase Parallel RLC Load  LConnTagsString=A|B|C  Configuration=Y (grounded)  NominalVoltage=Vphase_phase_lissage  Vabc=[1e3 1e3 1e3]  Vabcp=[1e3 1e3 1e3]  NominalFrequency=Freq  UnbalancedPower=off  ActivePower=P_lissage_min  InductivePower=0  CapacitivePower=0  Pabc=[10e3 9e3 11e3]  QLabc=[100 90 110]  QCabc=[100 90 110]  Pabcp=[10e3 9e3 11e3]  QLabcp=[100 90 110]  QCabcp=[100 90 110]  Measurements=None  LoadType=constant Z
      settings: SourceProductBaseCode=MT,PS
  Bit 1 : powerlib/Elements/Three-Phase Parallel RLC Load  LConnTagsString=A|B|C  Configuration=Y (grounded)  NominalVoltage=Vphase_phase_lissage  Vabc=[1e3 1e3 1e3]  Vabcp=[1e3 1e3 1e3]  NominalFrequency=Freq  UnbalancedPower=off  ActivePower=2*P_lissage_min  InductivePower=0  CapacitivePower=0  Pabc=[10e3 9e3 11e3]  QLabc=[100 90 110]  QCabc=[100 90 110]  Pabcp=[10e3 9e3 11e3]  QLabcp=[100 90 110]  QCabcp=[100 90 110]  Measurements=None  LoadType=constant Z
      settings: SourceProductBaseCode=MT,PS
  Bit 2 : powerlib/Elements/Three-Phase Parallel RLC Load  LConnTagsString=A|B|C  Configuration=Y (grounded)  NominalVoltage=Vphase_phase_lissage  Vabc=[1e3 1e3 1e3]  Vabcp=[1e3 1e3 1e3]  NominalFrequency=Freq  UnbalancedPower=off  ActivePower=2^2*P_lissage_min  InductivePower=0  CapacitivePower=0  Pabc=[10e3 9e3 11e3]  QLabc=[100 90 110]  QCabc=[100 90 110]  Pabcp=[10e3 9e3 11e3]  QLabcp=[100 90 110]  QCabcp=[100 90 110]  Measurements=None  LoadType=constant Z
      settings: SourceProductBaseCode=MT,PS
  Bit 3 : powerlib/Elements/Three-Phase Parallel RLC Load  LConnTagsString=A|B|C  Configuration=Y (grounded)  NominalVoltage=Vphase_phase_lissage  Vabc=[1e3 1e3 1e3]  Vabcp=[1e3 1e3 1e3]  NominalFrequency=Freq  UnbalancedPower=off  ActivePower=2^3*P_lissage_min  InductivePower=0  CapacitivePower=0  Pabc=[10e3 9e3 11e3]  QLabc=[100 90 110]  QCabc=[100 90 110]  Pabcp=[10e3 9e3 11e3]  QLabcp=[100 90 110]  QCabcp=[100 90 110]  Measurements=None  LoadType=constant Z
      settings: SourceProductBaseCode=MT,PS
  Bit 4 : powerlib/Elements/Three-Phase Parallel RLC Load  LConnTagsString=A|B|C  Configuration=Y (grounded)  NominalVoltage=Vphase_phase_lissage  Vabc=[1e3 1e3 1e3]  Vabcp=[1e3 1e3 1e3]  NominalFrequency=Freq  UnbalancedPower=off  ActivePower=2^4*P_lissage_min  InductivePower=0  CapacitivePower=0  Pabc=[10e3 9e3 11e3]  QLabc=[100 90 110]  QCabc=[100 90 110]  Pabcp=[10e3 9e3 11e3]  QLabcp=[100 90 110]  QCabcp=[100 90 110]  Measurements=None  LoadType=constant Z
      settings: SourceProductBaseCode=MT,PS
  Bit 5 : powerlib/Elements/Three-Phase Parallel RLC Load  LConnTagsString=A|B|C  Configuration=Y (grounded)  NominalVoltage=Vphase_phase_lissage  Vabc=[1e3 1e3 1e3]  Vabcp=[1e3 1e3 1e3]  NominalFrequency=Freq  UnbalancedPower=off  ActivePower=2^5*P_lissage_min  InductivePower=0  CapacitivePower=0  Pabc=[10e3 9e3 11e3]  QLabc=[100 90 110]  QCabc=[100 90 110]  Pabcp=[10e3 9e3 11e3]  QLabcp=[100 90 110]  QCabcp=[100 90 110]  Measurements=None  LoadType=constant Z
      settings: SourceProductBaseCode=MT,PS
  Bit 6 : powerlib/Elements/Three-Phase Parallel RLC Load  LConnTagsString=A|B|C  Configuration=Y (grounded)  NominalVoltage=Vphase_phase_lissage  Vabc=[1e3 1e3 1e3]  Vabcp=[1e3 1e3 1e3]  NominalFrequency=Freq  UnbalancedPower=off  ActivePower=2^6*P_lissage_min  InductivePower=0  CapacitivePower=0  Pabc=[10e3 9e3 11e3]  QLabc=[100 90 110]  QCabc=[100 90 110]  Pabcp=[10e3 9e3 11e3]  QLabcp=[100 90 110]  QCabcp=[100 90 110]  Measurements=None  LoadType=constant Z
      settings: SourceProductBaseCode=MT,PS
  Bit 7 : powerlib/Elements/Three-Phase Parallel RLC Load  LConnTagsString=A|B|C  Configuration=Y (grounded)  NominalVoltage=Vphase_phase_lissage  Vabc=[1e3 1e3 1e3]  Vabcp=[1e3 1e3 1e3]  NominalFrequency=Freq  UnbalancedPower=off  ActivePower=2^7*P_lissage_min  InductivePower=0  CapacitivePower=0  Pabc=[10e3 9e3 11e3]  QLabc=[100 90 110]  QCabc=[100 90 110]  Pabcp=[10e3 9e3 11e3]  QLabcp=[100 90 110]  QCabcp=[100 90 110]  Measurements=None  LoadType=constant Z
      settings: SourceProductBaseCode=MT,PS
  A0 : PMIOPort  Side=Left
  B0 : PMIOPort  Port=2  Side=Left
  C0 : PMIOPort  Port=3  Side=Left
  A1 : PMIOPort  Port=4  Side=Left
  B1 : PMIOPort  Port=5  Side=Left
  C1 : PMIOPort  Port=6  Side=Left
  A2 : PMIOPort  Port=7  Side=Left
  B2 : PMIOPort  Port=8  Side=Left
  C2 : PMIOPort  Port=9  Side=Left
  A3 : PMIOPort  Port=10  Side=Left
  B3 : PMIOPort  Port=11  Side=Left
  C3 : PMIOPort  Port=12  Side=Left
  A4 : PMIOPort  Port=13  Side=Left
  B4 : PMIOPort  Port=14  Side=Left
  C4 : PMIOPort  Port=15  Side=Left
  A5 : PMIOPort  Port=16  Side=Left
  B5 : PMIOPort  Port=17  Side=Left
  C5 : PMIOPort  Port=18  Side=Left
  A6 : PMIOPort  Port=19  Side=Left
  B6 : PMIOPort  Port=20  Side=Left
  C6 : PMIOPort  Port=21  Side=Left
  A7 : PMIOPort  Port=22  Side=Left
  B7 : PMIOPort  Port=23  Side=Left
  C7 : PMIOPort  Port=24  Side=Left
  connections:
  C7/RConn1 -- Bit 7/LConn3
  B7/RConn1 -- Bit 7/LConn2
  A7/RConn1 -- Bit 7/LConn1
  C6/RConn1 -- Bit 6/LConn3
  B6/RConn1 -- Bit 6/LConn2
  A6/RConn1 -- Bit 6/LConn1
  C5/RConn1 -- Bit 5/LConn3
  B5/RConn1 -- Bit 5/LConn2
  A5/RConn1 -- Bit 5/LConn1
  C4/RConn1 -- Bit 4/LConn3
  B4/RConn1 -- Bit 4/LConn2
  A4/RConn1 -- Bit 4/LConn1
  C3/RConn1 -- Bit 3/LConn3
  B3/RConn1 -- Bit 3/LConn2
  A3/RConn1 -- Bit 3/LConn1
  C2/RConn1 -- Bit 2/LConn3
  B2/RConn1 -- Bit 2/LConn2
  A2/RConn1 -- Bit 2/LConn1
  C1/RConn1 -- Bit 1/LConn3
  B1/RConn1 -- Bit 1/LConn2
  A1/RConn1 -- Bit 1/LConn1
  C0/RConn1 -- Bit 0/LConn3
  B0/RConn1 -- Bit 0/LConn2
  A0/RConn1 -- Bit 0/LConn1

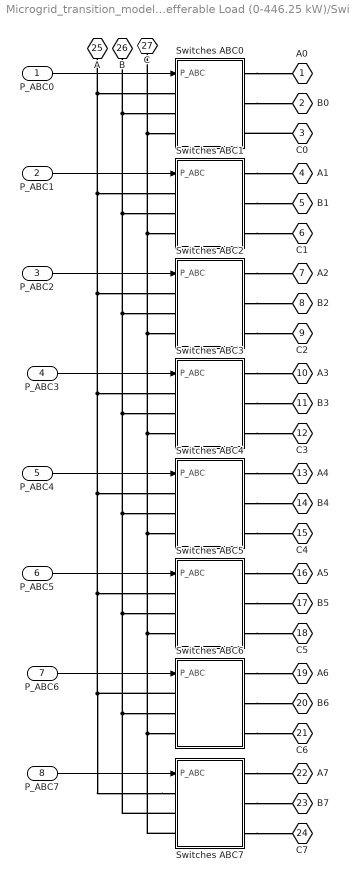
== system Microgrid_transition_model_092021/Defferable Load (0-446.25 kW)/Switches ==
  P_ABC0 : Inport
  P_ABC1 : Inport  Port=2
  P_ABC2 : Inport  Port=3
  P_ABC3 : Inport  Port=4
  P_ABC4 : Inport  Port=5
  P_ABC5 : Inport  Port=6
  P_ABC6 : Inport  Port=7
  P_ABC7 : Inport  Port=8
  Switches ABC0 : Subsystem
  Switches ABC1 : Subsystem
  Switches ABC2 : Subsystem
  Switches ABC3 : Subsystem
  Switches ABC4 : Subsystem
  Switches ABC5 : Subsystem
  Switches ABC6 : Subsystem
  Switches ABC7 : Subsystem
  A0 : PMIOPort  Side=Right
  B0 : PMIOPort  Port=2  Side=Right
  C0 : PMIOPort  Port=3  Side=Right
  A1 : PMIOPort  Port=4  Side=Right
  B1 : PMIOPort  Port=5  Side=Right
  C1 : PMIOPort  Port=6  Side=Right
  A2 : PMIOPort  Port=7  Side=Right
  B2 : PMIOPort  Port=8  Side=Right
  C2 : PMIOPort  Port=9  Side=Right
  A3 : PMIOPort  Port=10  Side=Right
  B3 : PMIOPort  Port=11  Side=Right
  C3 : PMIOPort  Port=12  Side=Right
  A4 : PMIOPort  Port=13  Side=Right
  B4 : PMIOPort  Port=14  Side=Right
  C4 : PMIOPort  Port=15  Side=Right
  A5 : PMIOPort  Port=16  Side=Right
  B5 : PMIOPort  Port=17  Side=Right
  C5 : PMIOPort  Port=18  Side=Right
  A6 : PMIOPort  Port=19  Side=Right
  B6 : PMIOPort  Port=20  Side=Right
  C6 : PMIOPort  Port=21  Side=Right
  A7 : PMIOPort  Port=22  Side=Right
  B7 : PMIOPort  Port=23  Side=Right
  C7 : PMIOPort  Port=24  Side=Right
  A : PMIOPort  Port=25  Side=Left
  B : PMIOPort  Port=26  Side=Left
  C : PMIOPort  Port=27  Side=Left
  wires:
  P_ABC7/1 -> Switches ABC7/1(P_ABC)
  P_ABC6/1 -> Switches ABC6/1(P_ABC)
  P_ABC5/1 -> Switches ABC5/1(P_ABC)
  P_ABC4/1 -> Switches ABC4/1(P_ABC)
  P_ABC3/1 -> Switches ABC3/1(P_ABC)
  P_ABC2/1 -> Switches ABC2/1(P_ABC)
  P_ABC1/1 -> Switches ABC1/1(P_ABC)
  P_ABC0/1 -> Switches ABC0/1(P_ABC)
  connections:
  Switches ABC0/RConn1 -- A0/RConn1
  Switches ABC0/RConn2 -- B0/RConn1
  C0/RConn1 -- Switches ABC0/RConn3
  Switches ABC1/RConn1 -- A1/RConn1
  Switches ABC1/RConn2 -- B1/RConn1
  Switches ABC1/RConn3 -- C1/RConn1
  Switches ABC2/RConn1 -- A2/RConn1
  Switches ABC2/RConn2 -- B2/RConn1
  Switches ABC2/RConn3 -- C2/RConn1
  Switches ABC3/RConn1 -- A3/RConn1
  Switches ABC3/RConn2 -- B3/RConn1
  Switches ABC3/RConn3 -- C3/RConn1
  Switches ABC4/RConn1 -- A4/RConn1
  Switches ABC4/RConn2 -- B4/RConn1
  Switches ABC4/RConn3 -- C4/RConn1
  Switches ABC5/RConn1 -- A5/RConn1
  Switches ABC5/RConn2 -- B5/RConn1
  Switches ABC5/RConn3 -- C5/RConn1
  Switches ABC6/RConn1 -- A6/RConn1
  Switches ABC6/RConn2 -- B6/RConn1
  Switches ABC6/RConn3 -- C6/RConn1
  Switches ABC7/RConn3 -- C7/RConn1
  Switches ABC7/RConn2 -- B7/RConn1
  Switches ABC7/RConn1 -- A7/RConn1
  Switches ABC7/LConn2 -- Switches ABC0/LConn2 -- B/RConn1 -- Switches ABC1/LConn2 -- Switches ABC2/LConn2 -- Switches ABC3/LConn2 -- Switches ABC4/LConn2 -- Switches ABC5/LConn2 -- Switches ABC6/LConn2
  Switches ABC7/LConn3 -- Switches ABC0/LConn3 -- C/RConn1 -- Switches ABC1/LConn3 -- Switches ABC2/LConn3 -- Switches ABC3/LConn3 -- Switches ABC4/LConn3 -- Switches ABC5/LConn3 -- Switches ABC6/LConn3
  Switches ABC7/LConn1 -- Switches ABC0/LConn1 -- A/RConn1 -- Switches ABC1/LConn1 -- Switches ABC2/LConn1 -- Switches ABC3/LConn1 -- Switches ABC4/LConn1 -- Switches ABC5/LConn1 -- Switches ABC6/LConn1

== system Microgrid_transition_model_092021/Discrete Frequency Regulator/Discrete PID Controller ==
  note: Pierre Giroux, Gilbert Sybille
      | Power System Simulation Laboratory
      | IREQ, Hydro-Quebc
  note: Discrete PID Controller
  Error : Inport  SampleTime=Ts
  "Derivative " : DiscreteTransferFcn  Numerator=[2 -2]  Denominator=[Ts+2*TcD Ts-2*TcD]  SampleTime=Ts
  Discrete-Time Integrator : DiscreteIntegrator  InitialCondition=Init  SampleTime=Ts  LimitOutput=on  UpperSaturationLimit=UpperLimit  LowerSaturationLimit=LowerLimit  ICPrevOutput=DiscIntNeverNeededParam  ICPrevScaledInput=DiscIntNeverNeededParam
  Kp4 : Gain  Gain=Kp  SaturateOnIntegerOverflow=on  SampleTime=Ts  OutDataTypeStr=Inherit: Same as input  ParamDataTypeStr=Inherit: Same as input
  Kp5 : Gain  Gain=Ki  SaturateOnIntegerOverflow=on  SampleTime=Ts  OutDataTypeStr=Inherit: Same as input  ParamDataTypeStr=Inherit: Same as input
  Kp6 : Gain  Gain=Kd  SaturateOnIntegerOverflow=on  SampleTime=Ts  OutDataTypeStr=Inherit: Same as input  ParamDataTypeStr=Inherit: Same as input
  Saturation2 : Saturate  UpperLimit=UpperLimit  LowerLimit=LowerLimit  SampleTime=Ts
  Sum6 : Sum  Inputs=+++  InputSameDT=on  SaturateOnIntegerOverflow=on  SampleTime=Ts  OutDataTypeStr=Inherit: Same as first input
  Zero-Order Hold : ZeroOrderHold  SampleTime=Ts
  Out : Outport  SampleTime=Ts  InitialOutput=0  VectorParamsAs1DForOutWhenUnconnected=off
  wires:
  Saturation2/1 -> Out/1
  Error/1 -> Kp4/1, Kp5/1, Kp6/1
  Sum6/1 -> Saturation2/1
  Kp5/1 -> Discrete-Time Integrator/1
  Kp6/1 -> "Derivative "/1
  Kp4/1 -> Zero-Order Hold/1
  Discrete-Time Integrator/1 -> Sum6/2
  "Derivative "/1 -> Sum6/3
  Zero-Order Hold/1 -> Sum6/1

== system Microgrid_transition_model_092021/Discrete Frequency Regulator/Pulses Decoder ==
  Code : Inport
  Constant : Constant  Value=pow2(0:-1:-(n-1))
  Constant6 : Constant  Value=2
  Math Function : Math  Operator=rem  SignedPower=on  SaturateOnIntegerOverflow=on
  Product : Product  InputSameDT=on  SaturateOnIntegerOverflow=on  OutDataTypeStr=Inherit: Same as first input
  Rounding Function : Rounding
  Pulses : Outport  VectorParamsAs1DForOutWhenUnconnected=off
  wires:
  Math Function/1 -> Pulses/1
  Rounding Function/1 -> Math Function/1
  Constant6/1 -> Math Function/2
  Product/1 -> Rounding Function/1
  Code/1 -> Product/1
  Constant/1 -> Product/2
